simulink model "CalculatAverage"  (R2021a)
settings: Solver=FixedStepAuto  StartTime=0.0  StopTime=10.0  RelTol=1e-3
settings Model: Creator=user  LastModifiedBy=user
settings OptimizationCC: DefaultParameterBehavior=Inlined  EnhancedBackFolding=on  PassReuseOutputArgsAs=Individual arguments  ZeroExternalMemoryAtStartup=off  ZeroInternalMemoryAtStartup=off  OptimizeBlockOrder=speed  DifferentSizesBufferReuse=on  OptimizationCustomize=off  EfficientTunableParamExpr=on
settings DebuggingCC: ParameterTunabilityLossMsg=error
settings SFSimCC: MATLABDynamicMemAlloc=off
settings RTWCC: SystemTargetFile=ert.tlc  GenCodeOnly=on  TemplateMakefile=ert_default_tmf  GenerateReport=on  IncludeHyperlinkInReport=on  LaunchReport=on  GenerateTraceInfo=on
settings CodeAppCC: ForceParamTrailComments=on  IgnoreCustomStorageClasses=off  OperatorAnnotations=on  SimulinkDataObjDesc=on  SFDataObjDesc=on  InsertBlockDesc=on
settings ERTTargetCC: TargetLangStandard=C99 (ISO)  GenerateSampleERTMain=on  InlinedParameterPlacement=NonHierarchical  ERTCustomFileTemplate=example_file_process.tlc

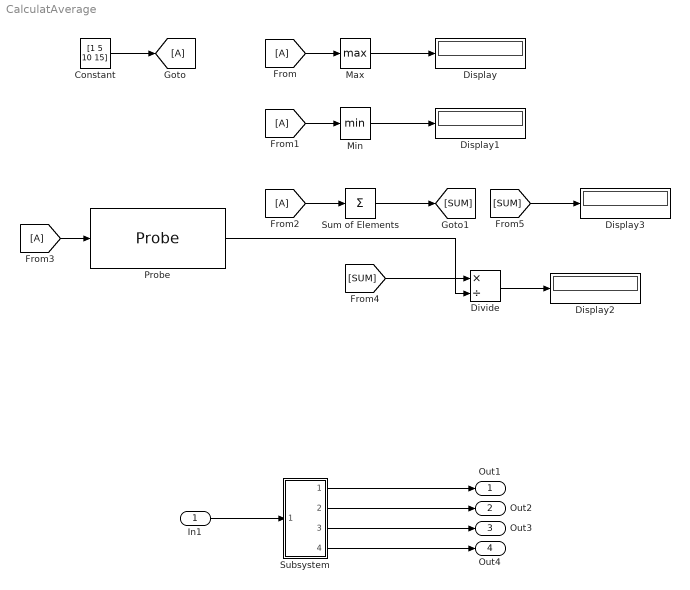
== system CalculatAverage ==
  In1 : Inport
  Constant : Constant  Value=[1 5 10 15]
  Display{,1..3} (4 alike) : Display
  Divide : Product  Inputs=*/
  Max : MinMax  Function=max
  Min : MinMax
  Probe : Probe  ProbeSampleTime=off  ProbeComplexSignal=off
  Subsystem : Subsystem
  Sum of Elements : Sum  Inputs=+
  Out1 : Outport
  Out2 : Outport  Port=2
  Out3 : Outport  Port=3
  Out4 : Outport  Port=4
  wires:
  Constant/1 -> [A]
  [A] -> Max/1
  [A] -> Min/1
  [A] -> Sum of Elements/1
  [A] -> Probe/1
  Sum of Elements/1 -> [SUM]
  [SUM] -> Divide/1
  Probe/1 -> Divide/2
  Max/1 -> Display/1
  Min/1 -> Display1/1
  Divide/1 -> Display2/1
  [SUM] -> Display3/1
  In1/1 -> Subsystem/1(In1)
  Subsystem/1(Out1) -> Out1/1
  Subsystem/2(Out2) -> Out2/1
  Subsystem/3(Out3) -> Out3/1
  Subsystem/4(Out4) -> Out4/1

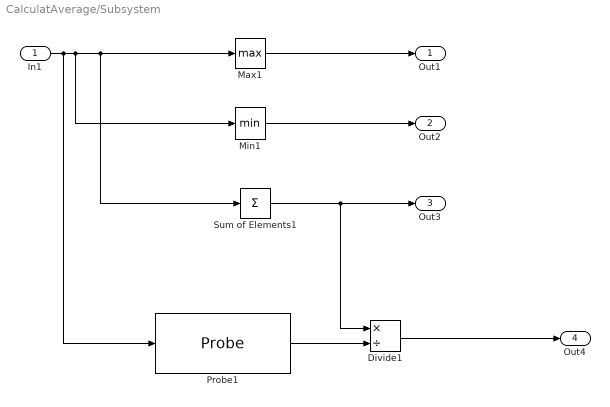
== system CalculatAverage/Subsystem ==
  In1 : Inport
  Divide1 : Product  Inputs=*/
  Max1 : MinMax  Function=max
  Min1 : MinMax
  Probe1 : Probe  ProbeSampleTime=off  ProbeComplexSignal=off
  Sum of Elements1 : Sum  Inputs=+
  Out1 : Outport
  Out2 : Outport  Port=2
  Out3 : Outport  Port=3
  Out4 : Outport  Port=4
  wires:
  Divide1/1 -> Out4/1
  In1/1 -> Probe1/1, Min1/1, Sum of Elements1/1, Max1/1
  Probe1/1 -> Divide1/2
  Min1/1 -> Out2/1
  Sum of Elements1/1 -> Out3/1, Divide1/1
  Max1/1 -> Out1/1
